simulink model "TEA_Ejercicios0_control_barco_Simulink"  (R2017b)
settings: Solver=ode4  StartTime=0.0  StopTime=300  FixedStep=1e-3  RelTol=1e-3
values from neighbouring files (symbols this model uses):
  beta = 2    [TEA_Ejercicios0_control_barco_sMatlab.m]    (also in lorentz.m = 2.66666666667; lorentzlqr.m = 2.66666666667)
  K = 0.12    [TEA_Ejercicios0_control_barco_sMatlab.m]
  Kact = 35/10    (= 3.5)    [TEA_Ejercicios0_control_barco_sMatlab.m]
  Kd2_y = ((alfa_y+2*xi)*wn*tau-1)/K3    (= 2657.98674525)    [TEA_Ejercicios0_control_barco_sMatlab.m]
  Kd_psi = (2*xi*wn*tau-1)/K2    (= 61.44)    [TEA_Ejercicios0_control_barco_sMatlab.m]
  Kd_r = 0    [TEA_Ejercicios0_control_barco_sMatlab.m]
  Kd_y = (2*xi*alfa_y+1)*tau*wn^2/K3    (= 221.478379034)    [TEA_Ejercicios0_control_barco_sMatlab.m]
  Ki_psi = 0    [TEA_Ejercicios0_control_barco_sMatlab.m]
  Ki_r = tau*wn^2/K1    (= 0.271172571429)    [TEA_Ejercicios0_control_barco_sMatlab.m]
  Ki_y = 0    [TEA_Ejercicios0_control_barco_sMatlab.m]
  Kp_psi = tau*wn^2/K2    (= 2.44055314286)    [TEA_Ejercicios0_control_barco_sMatlab.m]
  Kp_r = (2*xi*wn*tau-1)/K1    (= 6.82666666667)    [TEA_Ejercicios0_control_barco_sMatlab.m]
  Kp_y = alfa_y*wn^3*tau/K3    (= 4.71144915401)    [TEA_Ejercicios0_control_barco_sMatlab.m]
  tau = 26    [TEA_Ejercicios0_control_barco_sMatlab.m]    (also in ssoidentifica.m = 1.98491464867)
  tau_delta = 0.8    [TEA_Ejercicios0_control_barco_sMatlab.m]
  tau_fd = 0.05    [TEA_Ejercicios0_control_barco_sMatlab.m]
  V = 15*1852/3600    (= 7.71666666667)    [TEA_Ejercicios0_control_barco_sMatlab.m]
settings Model: Creator=USER  LastModifiedBy=pablo
settings DataIOCC: SaveFormat=StructureWithTime
settings OptimizationCC: LifeSpan=inf
settings DebuggingCC: SFExecutionAtInitializationDiag=none
settings HardwareCC: ProdBitPerSizeT=32  ProdBitPerPtrDiffT=32  ProdWordSize=32  ProdHWDeviceType=Specified
settings CodeAppCC: StateflowObjectComments=on

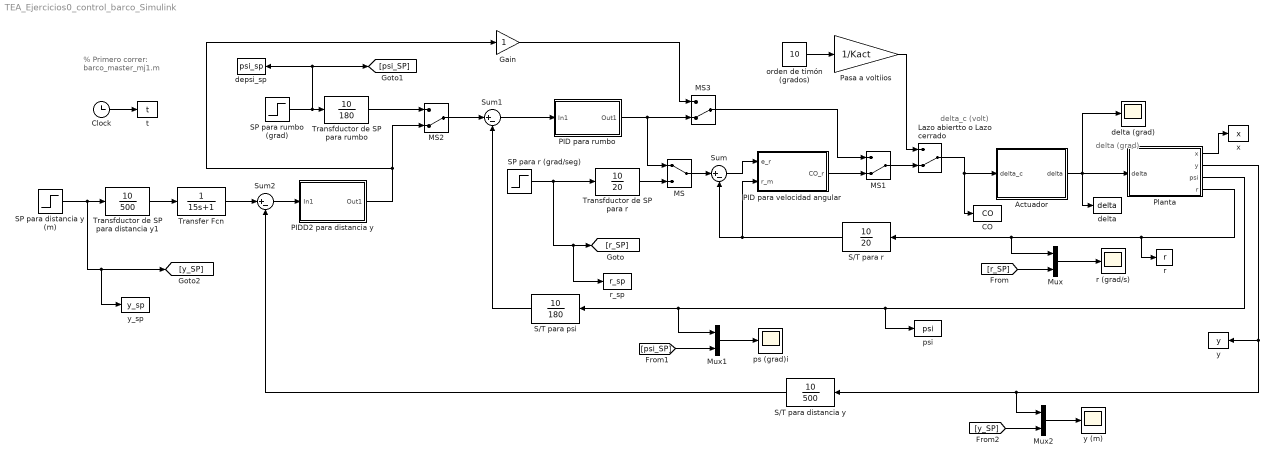
== system TEA_Ejercicios0_control_barco_Simulink ==
  note: % Primero correr:
      | barco_master_mj1.m
  note: delta_c
      | (volt)
  note: delta
      | (grad)
  " orden de timón (grados)" : Constant  Value=10
  Actuador : Subsystem
  CO : ToWorkspace  VariableName=CO  SampleTime=-1
  Clock : Clock
  Gain : Gain
  Lazo abiertto o Lazo cerrado : ManualSwitch  CurrentSetting=0
  MS : ManualSwitch
  MS1 : ManualSwitch  CurrentSetting=0
  MS2 : ManualSwitch  CurrentSetting=0
  MS3 : ManualSwitch  CurrentSetting=0
  Mux : Mux  Inputs=2
  Mux1 : Mux  Inputs=2
  Mux2 : Mux  Inputs=2
  PID para rumbo : Subsystem
  PID para velocidad angular : Subsystem
  PIDD2 para distancia y : Subsystem
  Pasa a voltiios : Gain  Gain=1/Kact
  Planta : Subsystem
  S/T para distancia y : TransferFcn  Numerator=[10]  Denominator=[500]
  S/T para psi : TransferFcn  Numerator=[10]  Denominator=[180]
  S/T para r : TransferFcn  Numerator=[10]  Denominator=[20]
  SP para distancia y (m) : Step  Time=10  After=100  SampleTime=0
  SP para r (grad/seg) : Step  After=0.5  SampleTime=0
  SP para rumbo (grad) : Step  Time=10  After=5  SampleTime=0
  Sum : Sum  Inputs=|+-
  Sum1 : Sum  Inputs=|+-
  Sum2 : Sum  Inputs=|+-
  Transfductor de SP para distancia y1 : TransferFcn  Numerator=[10]  Denominator=[500]
  Transfductor de SP para r : TransferFcn  Numerator=[10]  Denominator=[20]
  Transfductor de SP para rumbo : TransferFcn  Numerator=[10]  Denominator=[180]
  Transfer Fcn : TransferFcn  Denominator=[15 1]
  delta : ToWorkspace  VariableName=delta  SampleTime=-1
  delta (grad) : Scope
  depsi_sp : ToWorkspace  VariableName=psi_sp  SampleTime=-1
  ps (grad)i : Scope
  psi : ToWorkspace  VariableName=psi  SampleTime=-1
  r : ToWorkspace  VariableName=r  SampleTime=-1
  r (grad/s) : Scope
  r_sp : ToWorkspace  VariableName=r_sp  SampleTime=-1
  t : ToWorkspace  VariableName=t  SampleTime=-1
  x : ToWorkspace  VariableName=x  SampleTime=-1
  y : ToWorkspace  VariableName=y  SampleTime=-1
  y (m) : Scope
  y_sp : ToWorkspace  VariableName=y_sp  SampleTime=-1
  wires:
  Sum/1 -> PID para velocidad angular/1(e_r)
  S/T para r/1 -> PID para velocidad angular/2(r_m), Sum/2
  Sum1/1 -> PID para rumbo/1(In1)
  MS/1 -> Sum/1
  Transfductor de SP para r/1 -> MS/2
  PID para rumbo/1(Out1) -> MS3/2, MS/1
  SP para r (grad/seg)/1 -> r_sp/1, [r_SP], Transfductor de SP para r/1
  S/T para psi/1 -> Sum1/2
  PID para velocidad angular/1(CO_r) -> MS1/2
  SP para rumbo (grad)/1 -> depsi_sp/1, [psi_SP], Transfductor de SP para rumbo/1
  Sum2/1 -> PIDD2 para distancia y/1(In1)
  Transfductor de SP para distancia y1/1 -> Transfer Fcn/1
  S/T para distancia y/1 -> Sum2/2
  MS2/1 -> Sum1/1
  Planta/4(r) -> r/1, Mux/1, S/T para r/1
  Planta/3(psi) -> psi/1, Mux1/1, S/T para psi/1
  Actuador/1(delta) -> delta/1, delta (grad)/1, Planta/1(delta)
  Mux/1 -> r (grad/s)/1
  [r_SP] -> Mux/2
  Mux1/1 -> ps (grad)i/1
  [psi_SP] -> Mux1/2
  PIDD2 para distancia y/1(Out1) -> Gain/1, MS2/2
  Transfductor de SP para rumbo/1 -> MS2/1
  Gain/1 -> MS3/1
  MS3/1 -> MS1/1
  [y_SP] -> Mux2/2
  Mux2/1 -> y (m)/1
  SP para distancia y (m)/1 -> y_sp/1, [y_SP], Transfductor de SP para distancia y1/1
  Transfer Fcn/1 -> Sum2/1
  Planta/2(y) -> y/1, Mux2/1, S/T para distancia y/1
  Planta/1(x) -> x/1
  MS1/1 -> Lazo abiertto o Lazo cerrado/2
  Lazo abiertto o Lazo cerrado/1 -> CO/1, Actuador/1(delta_c)
  " orden de timón (grados)"/1 -> Pasa a voltiios/1
  Pasa a voltiios/1 -> Lazo abiertto o Lazo cerrado/1
  Clock/1 -> t/1

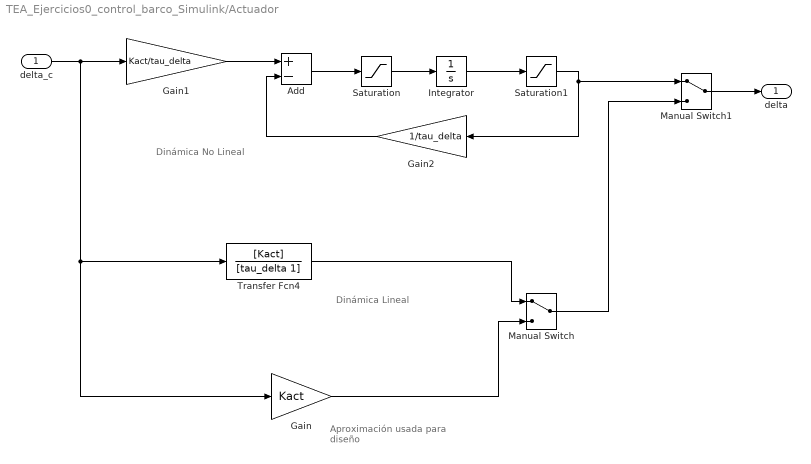
== system TEA_Ejercicios0_control_barco_Simulink/Actuador ==
  note: Aproximación usada
      | para diseño
  note: Dinámica Lineal
  note: Dinámica No Lineal
  delta_c : Inport
  Add : Sum  Inputs=+-
  Gain : Gain  Gain=Kact
  Gain1 : Gain  Gain=Kact/tau_delta
  Gain2 : Gain  Gain=1/tau_delta
  Integrator : Integrator
  Manual Switch : ManualSwitch
  Manual Switch1 : ManualSwitch
  Saturation : Saturate  UpperLimit=8  LowerLimit=-8
  Saturation1 : Saturate  UpperLimit=35  LowerLimit=-35
  Transfer Fcn4 : TransferFcn  Numerator=[Kact]  Denominator=[tau_delta 1]
  delta : Outport
  wires:
  Transfer Fcn4/1 -> Manual Switch/1
  Gain/1 -> Manual Switch/2
  delta_c/1 -> Gain1/1, Gain/1, Transfer Fcn4/1
  Gain1/1 -> Add/1
  Add/1 -> Saturation/1
  Saturation/1 -> Integrator/1
  Integrator/1 -> Saturation1/1
  Saturation1/1 -> Manual Switch1/1, Gain2/1
  Manual Switch/1 -> Manual Switch1/2
  Manual Switch1/1 -> delta/1
  Gain2/1 -> Add/2

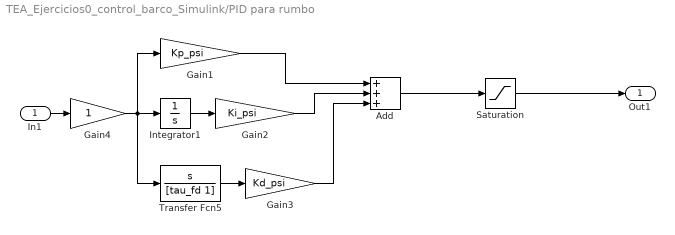
== system TEA_Ejercicios0_control_barco_Simulink/PID para rumbo ==
  In1 : Inport
  Add : Sum  Inputs=+++
  Gain1 : Gain  Gain=Kp_psi
  Gain2 : Gain  Gain=Ki_psi
  Gain3 : Gain  Gain=Kd_psi
  Gain4 : Gain
  Integrator1 : Integrator
  Saturation : Saturate  UpperLimit=10  LowerLimit=-10
  Transfer Fcn5 : TransferFcn  Numerator="[1  0]"  Denominator=[tau_fd 1]
  Out1 : Outport
  wires:
  In1/1 -> Gain4/1
  Gain3/1 -> Add/3
  Add/1 -> Saturation/1
  Transfer Fcn5/1 -> Gain3/1
  Gain1/1 -> Add/1
  Integrator1/1 -> Gain2/1
  Gain2/1 -> Add/2
  Gain4/1 -> Transfer Fcn5/1, Gain1/1, Integrator1/1
  Saturation/1 -> Out1/1

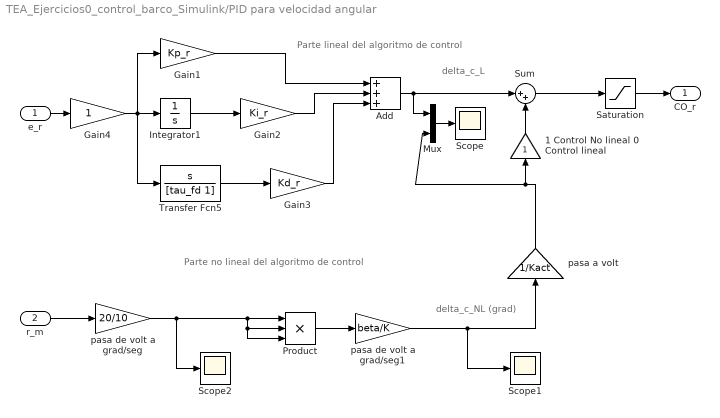
== system TEA_Ejercicios0_control_barco_Simulink/PID para velocidad angular ==
  note: Parte lineal del algoritmo de control
  note: Parte no lineal del algoritmo de control
  note: delta_c_NL (grad)
  note: delta_c_L
  e_r : Inport
  r_m : Inport  Port=2
  1 Control No lineal 0 Control lineal : Gain
  Add : Sum  Inputs=+++
  Gain1 : Gain  Gain=Kp_r
  Gain2 : Gain  Gain=Ki_r
  Gain3 : Gain  Gain=Kd_r
  Gain4 : Gain
  Integrator1 : Integrator
  Mux : Mux  Inputs=2
  Product : Product  Inputs=3
  Saturation : Saturate  UpperLimit=10  LowerLimit=-10
  Scope : Scope
  Scope1 : Scope
  Scope2 : Scope
  Sum : Sum  Inputs=|++
  Transfer Fcn5 : TransferFcn  Numerator="[1  0]"  Denominator=[tau_fd 1]
  pasa a volt : Gain  Gain=1/Kact
  pasa de volt a grad/seg : Gain  Gain=20/10
  pasa de volt a grad/seg1 : Gain  Gain=beta/K
  CO_r : Outport
  wires:
  e_r/1 -> Gain4/1
  Gain3/1 -> Add/3
  Transfer Fcn5/1 -> Gain3/1
  Gain1/1 -> Add/1
  Integrator1/1 -> Gain2/1
  Gain2/1 -> Add/2
  Gain4/1 -> Transfer Fcn5/1, Gain1/1, Integrator1/1
  Saturation/1 -> CO_r/1
  r_m/1 -> pasa de volt a grad/seg/1
  pasa de volt a grad/seg/1 -> Product/3, Product/2, Product/1, Scope2/1
  Product/1 -> pasa de volt a grad/seg1/1
  pasa de volt a grad/seg1/1 -> Scope1/1, pasa a volt/1
  Add/1 -> Mux/1, Sum/1
  Sum/1 -> Saturation/1
  1 Control No lineal 0 Control lineal/1 -> Sum/2
  Mux/1 -> Scope/1
  pasa a volt/1 -> Mux/2, 1 Control No lineal 0 Control lineal/1

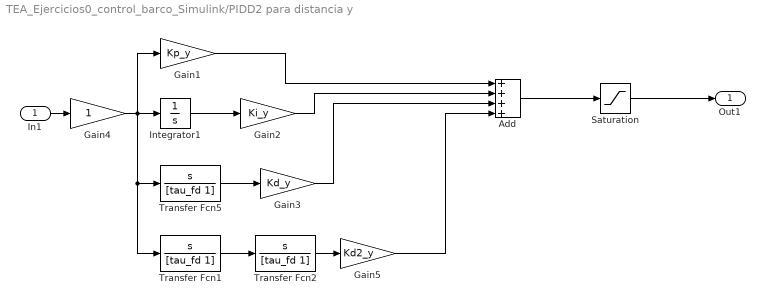
== system TEA_Ejercicios0_control_barco_Simulink/PIDD2 para distancia y ==
  In1 : Inport
  Add : Sum  Inputs=++++
  Gain1 : Gain  Gain=Kp_y
  Gain2 : Gain  Gain=Ki_y
  Gain3 : Gain  Gain=Kd_y
  Gain4 : Gain
  Gain5 : Gain  Gain=Kd2_y
  Integrator1 : Integrator
  Saturation : Saturate  UpperLimit=10  LowerLimit=-10
  Transfer Fcn1 : TransferFcn  Numerator="[1  0]"  Denominator=[tau_fd 1]
  Transfer Fcn2 : TransferFcn  Numerator="[1  0]"  Denominator=[tau_fd 1]
  Transfer Fcn5 : TransferFcn  Numerator="[1  0]"  Denominator=[tau_fd 1]
  Out1 : Outport
  wires:
  In1/1 -> Gain4/1
  Gain3/1 -> Add/3
  Add/1 -> Saturation/1
  Transfer Fcn5/1 -> Gain3/1
  Gain1/1 -> Add/1
  Integrator1/1 -> Gain2/1
  Gain2/1 -> Add/2
  Gain4/1 -> Transfer Fcn1/1, Transfer Fcn5/1, Gain1/1, Integrator1/1
  Transfer Fcn1/1 -> Transfer Fcn2/1
  Transfer Fcn2/1 -> Gain5/1
  Gain5/1 -> Add/4
  Saturation/1 -> Out1/1

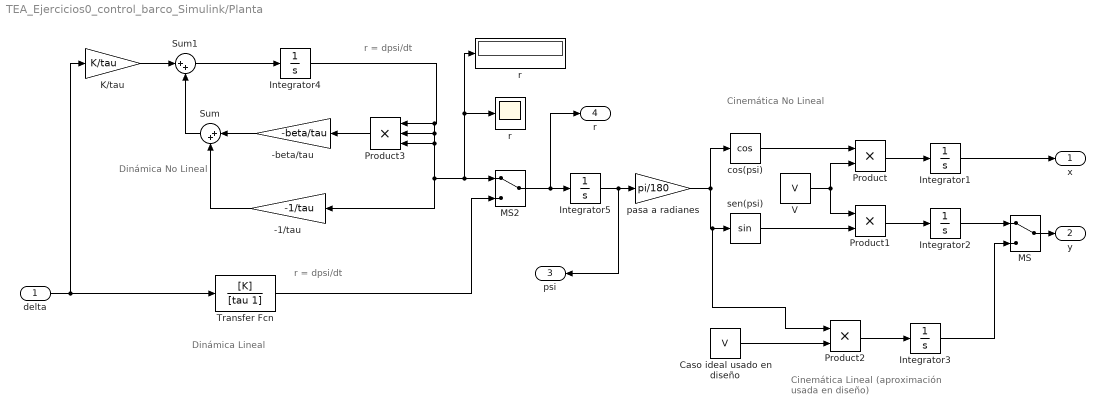
== system TEA_Ejercicios0_control_barco_Simulink/Planta ==
  note: Cinemática Lineal
      | (aproximación usada en diseño)
  note: Cinemática No Lineal
  note: Dinámica Lineal
  note: Dinámica
      | No Lineal
  note: r = dpsi/dt
  note: r = dpsi/dt
  delta : Inport
  "  r  " : Scope
  " MS   " : ManualSwitch
  " cos(psi)" : Trigonometry  Operator=cos
  " r " : Display
  -1/tau : Gain  Gain=-1/tau
  -beta/tau : Gain  Gain=-beta/tau
  Caso ideal usado en diseño : Constant  Value=V
  Integrator{1..5} (5 alike) : Integrator
  K/tau : Gain  Gain=K/tau
  MS2 : ManualSwitch
  Product : Product
  Product1 : Product
  Product2 : Product
  Product3 : Product  Inputs=3
  Sum : Sum  Inputs=|++
  Sum1 : Sum  Inputs=|++
  Transfer Fcn : TransferFcn  Numerator=[K]  Denominator=[tau 1]
  V : Constant  Value=V
  pasa a radianes : Gain  Gain=pi/180
  sen(psi) : Trigonometry
  x : Outport
  y : Outport  Port=2
  psi : Outport  Port=3
  r : Outport  Port=4
  wires:
  Transfer Fcn/1 -> MS2/2
  Product3/1 -> -beta/tau/1
  -beta/tau/1 -> Sum/1
  -1/tau/1 -> Sum/2
  K/tau/1 -> Sum1/1
  Sum/1 -> Sum1/2
  Sum1/1 -> Integrator4/1
  sen(psi)/1 -> Product1/2
  Product/1 -> Integrator1/1
  Product1/1 -> Integrator2/1
  pasa a radianes/1 -> Product2/1, sen(psi)/1, " cos(psi)"/1
  V/1 -> Product1/1, Product/2
  " cos(psi)"/1 -> Product/1
  Integrator1/1 -> x/1
  Caso ideal usado en diseño/1 -> Product2/2
  Product2/1 -> Integrator3/1
  Integrator3/1 -> " MS   "/2
  Integrator2/1 -> " MS   "/1
  " MS   "/1 -> y/1
  Integrator4/1 -> -1/tau/1, " r "/1, "  r  "/1, MS2/1, Product3/3, Product3/2, Product3/1
  MS2/1 -> r/1, Integrator5/1
  Integrator5/1 -> psi/1, pasa a radianes/1
  delta/1 -> K/tau/1, Transfer Fcn/1
